simulink model "boostconverter"  (R2017b)
settings: Solver=VariableStepAuto  StartTime=0.0  StopTime=5  MaxStep=1e-4  RelTol=1e-3
undefined symbols (not defined in the file): Imag, Real
libraries: powerlib x10, simulink x2, pePwmGenerator x1
settings Model: Creator=Orhun  LastModifiedBy=Orhun
settings DebuggingCC: AlgebraicLoopMsg=none  ArtificialAlgebraicLoopMsg=none

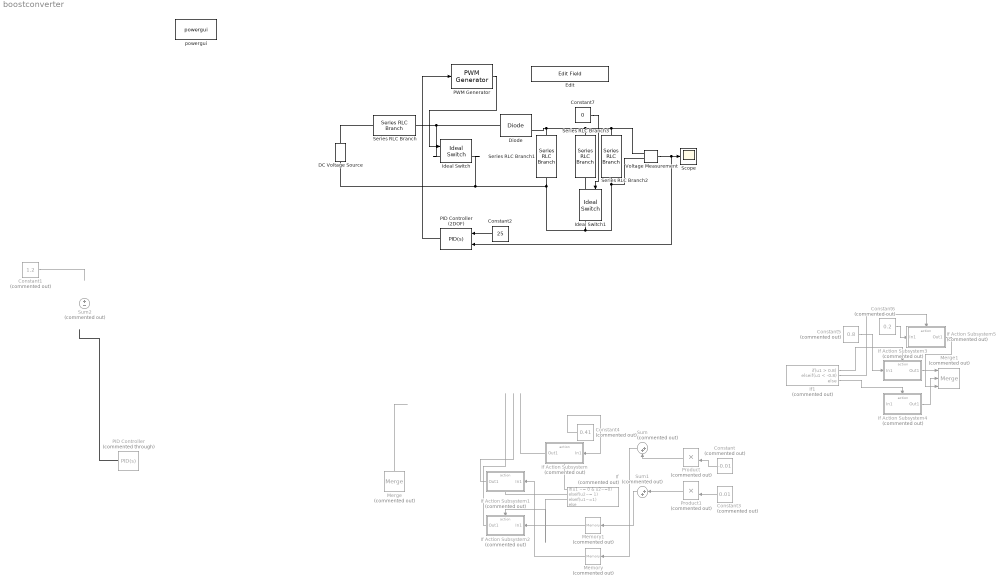
== system boostconverter ==
  Constant : Constant  Commented=on  Value=-0.01
  Constant1 : Constant  Commented=on  Value=1.2
  Constant2 : Constant  Value=25
  Constant3 : Constant  Commented=on  Value=0.01
  Constant4 : Constant  Commented=on  Value=0.41
  Constant5 : Constant  Commented=on  Value=0.8
  Constant6 : Constant  Commented=on  Value=0.2
  Constant7 : Constant  Value=0
  DC Voltage Source : powerlib/Electrical Sources/DC Voltage Source  Amplitude=15  Measurements=None
  Diode : powerlib/Power Electronics/Diode  Ron=0.001  Lon=0  Vf=0  IC=0  UseSnubber=0  Rs=0  Cs=0  Measurements=on
  Edit : EditField  WebBlockId=109  ModelName=boostconverter  LabelPosition=Hide  ShowInitialText=off  Alignment=Center
  Ideal Switch : powerlib/Power Electronics/Ideal Switch  Ron=0  Lon=0  IC=0  Rs=inf  Cs=inf  Measurements=on
  Ideal Switch1 : powerlib/Power Electronics/Ideal Switch  Ron=0.0001  Lon=0  IC=0  Rs=inf  Cs=inf  Measurements=on
  If : If  Commented=on  NumInputs=2  IfExpression=u1 ~= 0 & u2~=0  ElseIfExpressions=u2~= 1 , u1~=1
  If Action Subsystem : Subsystem  Commented=on  TreatAsAtomicUnit=on
  If Action Subsystem1 : Subsystem  Commented=on  TreatAsAtomicUnit=on
  If Action Subsystem2 : Subsystem  Commented=on  TreatAsAtomicUnit=on
  If Action Subsystem3 : Subsystem  Commented=on  TreatAsAtomicUnit=on
  If Action Subsystem4 : Subsystem  Commented=on  TreatAsAtomicUnit=on
  If Action Subsystem5 : Subsystem  Commented=on  TreatAsAtomicUnit=on
  If1 : If  Commented=on  IfExpression=u1 > 0.8  ElseIfExpressions=u1 < -0.8
  Memory : Memory  Commented=on  InitialCondition=0.41
  Memory1 : Memory  Commented=on  InitialCondition=0.41
  Merge : Merge  Commented=on  Inputs=3  InitialOutput=0.4
  Merge1 : Merge  Commented=on  Inputs=3  InitialOutput=0.4
  PID Controller : simulink/Continuous/PID Controller  Commented=through  Controller=PID  TimeDomain=Continuous-time  SampleTime=-1  IntegratorMethod=Forward Euler  FilterMethod=Forward Euler  Form=Parallel  UseFilter=on  ControllerParametersSource=internal  P=0.026  I=0.000005  D=0.00005  N=100  InitialConditionSource=internal  InitialConditionForIntegrator=0  InitialConditionForFilter=0  ExternalReset=none  LimitOutput=on  UpperSaturationLimit=0.77  LowerSaturationLimit=0.3  LinearizeAsGain=on  AntiWindupMode=none  Kb=1  TrackingMode=off  Kt=1  PParamMin=[]  PParamMax=[]  IParamMin=[]  IParamMax=[]  DParamMin=[]  DParamMax=[]  NParamMin=[]  NParamMax=[]  KbParamMin=[]  KbParamMax=[]  KtParamMin=[]  KtParamMax=[]  POutMin=[]  POutMax=[]  IOutMin=[]  IOutMax=[]  DOutMin=[]  DOutMax=[]  NOutMin=[]  NOutMax=[]  KbOutMin=[]  KbOutMax=[]  KtOutMin=[]  KtOutMax=[]  IntegratorOutMin=[]  IntegratorOutMax=[]  FilterOutMin=[]  FilterOutMax=[]  SumOutMin=[]  SumOutMax=[]  SumI1OutMin=[]  SumI1OutMax=[]  SumI2OutMin=[]  SumI2OutMax=[]  SumI3OutMin=[]  SumI3OutMax=[]  SumDOutMin=[]  SumDOutMax=[]  SaturationOutMin=[]  SaturationOutMax=[]  IntegratorContinuousStateAttributes=''  IntegratorStateMustResolveToSignalObject=off  IntegratorRTWStateStorageClass=Auto  FilterContinuousStateAttributes=''  FilterStateMustResolveToSignalObject=off  FilterRTWStateStorageClass=Auto  DifferentiatorICPrevScaledInput=0  DifferentiatorOutMin=[]  DifferentiatorOutMax=[]  InitialConditionSetting=State (most efficient)  FilterDiffOutCoefMin=[]  FilterDiffOutCoefMax=[]  SumDenOutMin=[]  SumDenOutMax=[]  SumNumOutMin=[]  SumNumOutMax=[]  ReciprocalOutMin=[]  ReciprocalOutMax=[]  DivideOutMin=[]  DivideOutMax=[]  TunerSelectOption=Transfer Function Based (PID Tuner App)
  PID Controller (2DOF) : simulink/Continuous/PID Controller (2DOF)  Controller=PID  TimeDomain=Continuous-time  SampleTime=-1  IntegratorMethod=Forward Euler  FilterMethod=Forward Euler  Form=Parallel  UseFilter=on  ControllerParametersSource=internal  P=0.065  I=20  D=0.0007  N=100  b=1  c=1  InitialConditionSource=internal  InitialConditionForIntegrator=0  InitialConditionForFilter=0  ExternalReset=none  LimitOutput=on  UpperSaturationLimit=1  LowerSaturationLimit=0.1  LinearizeAsGain=on  AntiWindupMode=none  Kb=1  TrackingMode=off  Kt=1  PParamMin=[]  PParamMax=[]  IParamMin=[]  IParamMax=[]  DParamMin=[]  DParamMax=[]  NParamMin=[]  NParamMax=[]  bParamMin=[]  bParamMax=[]  cParamMin=[]  cParamMax=[]  KbParamMin=[]  KbParamMax=[]  KtParamMin=[]  KtParamMax=[]  POutMin=[]  POutMax=[]  IOutMin=[]  IOutMax=[]  DOutMin=[]  DOutMax=[]  NOutMin=[]  NOutMax=[]  bOutMin=[]  bOutMax=[]  cOutMin=[]  cOutMax=[]  KbOutMin=[]  KbOutMax=[]  KtOutMin=[]  KtOutMax=[]  IntegratorOutMin=[]  IntegratorOutMax=[]  FilterOutMin=[]  FilterOutMax=[]  SumOutMin=[]  SumOutMax=[]  Sum1OutMin=[]  Sum1OutMax=[]  Sum2OutMin=[]  Sum2OutMax=[]  Sum3OutMin=[]  Sum3OutMax=[]  SumI1OutMin=[]  SumI1OutMax=[]  SumI2OutMin=[]  SumI2OutMax=[]  SumI3OutMin=[]  SumI3OutMax=[]  SumDOutMin=[]  SumDOutMax=[]  SaturationOutMin=[]  SaturationOutMax=[]  IntegratorContinuousStateAttributes=''  IntegratorStateMustResolveToSignalObject=off  IntegratorRTWStateStorageClass=Auto  FilterContinuousStateAttributes=''  FilterStateMustResolveToSignalObject=off  FilterRTWStateStorageClass=Auto  DifferentiatorICPrevScaledInput=0  DifferentiatorOutMin=[]  DifferentiatorOutMax=[]  InitialConditionSetting=State (most efficient)  FilterDiffOutCoefMin=[]  FilterDiffOutCoefMax=[]  SumDenOutMin=[]  SumDenOutMax=[]  SumNumOutMin=[]  SumNumOutMax=[]  ReciprocalOutMin=[]  ReciprocalOutMax=[]  DivideOutMin=[]  DivideOutMax=[]  TunerSelectOption=Transfer Function Based (PID Tuner App)
  PWM Generator : pePwmGenerator/PWM Generator  CarrCount=Up  Tper=5e-6  Ts=1e-7
  Product : Product  Commented=on
  Product1 : Product  Commented=on
  Scope : Scope
  Series RLC Branch : powerlib/Elements/Series RLC Branch  LConnTagsString=__new0  RConnTagsString=__new0  BranchType=L  Resistance=0  Inductance=5e-5  SetiL0=off  InitialCurrent=0  Capacitance=0  Setx0=off  InitialVoltage=0  Measurements=None
  Series RLC Branch1 : powerlib/Elements/Series RLC Branch  LConnTagsString=__new0  RConnTagsString=__new0  BranchType=C  Resistance=1  Inductance=1e-3  SetiL0=off  InitialCurrent=0  Capacitance=47e-6  Setx0=off  InitialVoltage=0  Measurements=None
  Series RLC Branch2 : powerlib/Elements/Series RLC Branch  LConnTagsString=__new0  RConnTagsString=__new0  BranchType=R  Resistance=12.5  Inductance=1e-3  SetiL0=off  InitialCurrent=0  Capacitance=1e-6  Setx0=off  InitialVoltage=0  Measurements=None
  Series RLC Branch3 : powerlib/Elements/Series RLC Branch  LConnTagsString=__new0  RConnTagsString=__new0  BranchType=R  Resistance=8.83  Inductance=1e-3  SetiL0=off  InitialCurrent=0  Capacitance=1e-6  Setx0=off  InitialVoltage=0  Measurements=None
  Sum : Sum  Commented=on  Inputs=|++
  Sum1 : Sum  Commented=on  Inputs=|++
  Sum2 : Sum  Commented=on  Inputs=+-
  Voltage Measurement : powerlib/Measurements/Voltage Measurement  PhasorSimulation=off  OutputType=Real-Imag  PSBequivalent=0
  powergui : powerlib/powergui  Priority=1  SimulationMode=Continuous  SampleTime=50e-6  frequency=60  Iterations=50  frequencyindice=0  Pbase=100e6  ErrMax=1e-4  UnitsV=kV  UnitsW=MW  buscounter=0  FunctionMessages=off  echomessages=off  EnableUseOfTLC=off  CurrentSourceSwitches=off  DisableSnubberDevices=off  DisableRonSwitches=off  DisableVfSwitches=off  DisplayEquations=off  SolverType=Tustin/Backward Euler (TBE)  Interpol=off  ExternalGateDelay=off  methode=off  Ts=100  x0status=blocks  SPID=on  SwTol=0  HookPort=off  RestoreLinks=warning  ResistiveCurrentMeasurement=off  Frange=[0:2:500]  Ylog=off  Xlog=on  ShowGrid=off  save=off  variable=ZData  structure=0  ZoomFFT=off  StartTime=0.0  cycles=1  DisplayStyle=1  fundamental=60  FreqAxis=off  MaxFrequency=1000  frequencyindicesteady=1  RmsSteady=1  display=off
  wires:
  PWM Generator/1 -> Ideal Switch/1
  Voltage Measurement/1 -> PID Controller (2DOF)/2, Scope/1
  Merge/1 -> ?
  If Action Subsystem3/1(Out1) -> Merge1/1
  Constant5/1 -> If Action Subsystem3/1(In1)
  If Action Subsystem4/1(Out1) -> Merge1/2
  If1/1 -> If Action Subsystem3/Action
  Constant6/1 -> If Action Subsystem5/1(In1)
  If1/3 -> If Action Subsystem4/Action
  ? -> If Action Subsystem4/1(In1)
  If Action Subsystem5/1(Out1) -> Merge1/3
  If1/2 -> If Action Subsystem5/Action
  ? -> If/1, Product/1
  ? -> Sum1/2, Sum/1
  Memory1/1 -> If Action Subsystem2/1(In1)
  Sum/1 -> Memory/1
  If Action Subsystem/1(Out1) -> ?
  Product1/1 -> Sum1/1
  Product/1 -> Sum/2
  ? -> Product1/1
  If Action Subsystem1/1(Out1) -> ?
  If/3 -> If Action Subsystem2/Action
  If Action Subsystem2/1(Out1) -> ?
  Constant4/1 -> If Action Subsystem/1(In1)
  ? -> If/2
  Sum1/1 -> Memory1/1
  If/1 -> If Action Subsystem/Action
  If/2 -> If Action Subsystem1/Action
  Constant3/1 -> Product1/2
  Constant/1 -> Product/2
  Memory/1 -> If Action Subsystem1/1(In1)
  Constant1/1 -> ?
  PID Controller/1 -> ?
  Constant2/1 -> PID Controller (2DOF)/1
  PID Controller (2DOF)/1 -> PWM Generator/1
  Constant7/1 -> Ideal Switch1/1
  connections:
  DC Voltage Source/RConn1 -- Series RLC Branch/LConn1
  Diode/LConn1 -- Ideal Switch/LConn1 -- Series RLC Branch/RConn1
  Ideal Switch1/RConn1 -- Voltage Measurement/LConn2 -- Series RLC Branch2/RConn1 -- Series RLC Branch1/RConn1 -- Ideal Switch/RConn1 -- DC Voltage Source/LConn1
  Series RLC Branch2/LConn1 -- Voltage Measurement/LConn1 -- Diode/RConn1 -- Series RLC Branch1/LConn1 -- Series RLC Branch3/LConn1
  Ideal Switch1/LConn1 -- Series RLC Branch3/RConn1

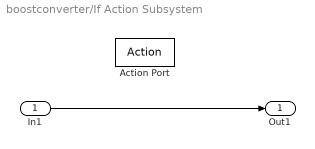
== system boostconverter/If Action Subsystem ==
  In1 : Inport
  Action Port : ActionPort  ActionType=then
  Out1 : Outport
  wires:
  In1/1 -> Out1/1

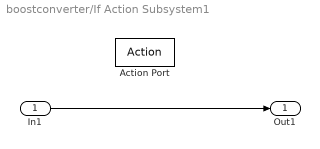
== system boostconverter/If Action Subsystem1 ==
  In1 : Inport
  Action Port : ActionPort  ActionType=elseif
  Out1 : Outport
  wires:
  In1/1 -> Out1/1

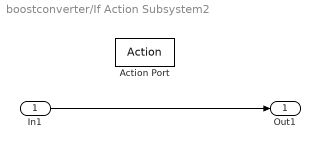
== system boostconverter/If Action Subsystem2 ==
  In1 : Inport
  Action Port : ActionPort  ActionType=elseif
  Out1 : Outport
  wires:
  In1/1 -> Out1/1

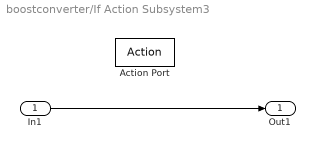
== system boostconverter/If Action Subsystem3 ==
  In1 : Inport
  Action Port : ActionPort  ActionType=then
  Out1 : Outport
  wires:
  In1/1 -> Out1/1

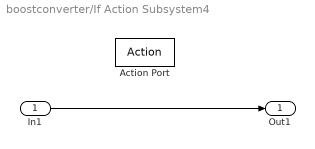
== system boostconverter/If Action Subsystem4 ==
  In1 : Inport
  Action Port : ActionPort  ActionType=else
  Out1 : Outport
  wires:
  In1/1 -> Out1/1

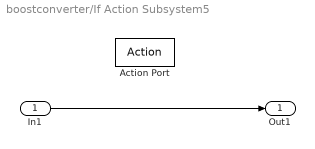
== system boostconverter/If Action Subsystem5 ==
  In1 : Inport
  Action Port : ActionPort  ActionType=elseif
  Out1 : Outport
  wires:
  In1/1 -> Out1/1
